simulink model "stm32f0_ccp_sensor"  (Simulink 7.3)
settings: Solver=ode3  SolverMode=SingleTasking  StartTime=0.0  StopTime=10.0  RelTol=1e-3
PreLoadFcn:
  | waijung.modelPreload; % Required for working with Waijung Blockset. Do not remove.
undefined symbols (not defined in the file): ARM, LQFP48, MDK, STM32F072CB
libraries: simulink x216, waijung_soft_i2c_lib x28, waijung_addon_module x12, stm32f0_flash_lib x10, stm32f0_can_lib x3, stm32f0_reset_lib x1, waijung_crc_lib x1, stm32f0_boot_lib x1, stm32f0_device_config_lib x1
(part 3 of 6)

== system stm32f0_ccp_sensor/HIH6131/Read/Subsystem ==
  In1 : Inport
  Enable : EnablePort
  Bitwise Operator : simulink/Logic and Bit Operations/Bitwise Operator  logicop=OR  UseBitMask=off  NumInputPorts=2  BitMask=bin2dec('11011001')  BitMaskRealWorld=Stored Integer
  Bitwise Operator1 : simulink/Logic and Bit Operations/Bitwise Operator  logicop=OR  UseBitMask=off  NumInputPorts=2  BitMask=bin2dec('11011001')  BitMaskRealWorld=Stored Integer
  Bitwise Operator2 : simulink/Logic and Bit Operations/Bitwise Operator  logicop=AND  UseBitMask=on  BitMask=hex2dec('3FFF')  BitMaskRealWorld=Stored Integer
  Bitwise Operator3 : simulink/Logic and Bit Operations/Bitwise Operator  logicop=AND  UseBitMask=on  BitMask=hex2dec('C000')  BitMaskRealWorld=Stored Integer
  Data Type Conversion : DataTypeConversion  OutDataTypeMode=uint16  OutDataType=fixdt(1, 16)  OutScaling=2^0  OutDataTypeStr=uint16
  Demux : Demux
  Shift Arithmetic : simulink/Logic and Bit Operations/Shift Arithmetic  SystemSampleTime=-1  nBitShiftRight=-8  nBinPtShiftRight=0
  Shift Arithmetic1 : simulink/Logic and Bit Operations/Shift Arithmetic  SystemSampleTime=-1  nBitShiftRight=-8  nBinPtShiftRight=0
  Shift Arithmetic2 : simulink/Logic and Bit Operations/Shift Arithmetic  SystemSampleTime=-1  nBitShiftRight=2  nBinPtShiftRight=0
  Shift Arithmetic3 : simulink/Logic and Bit Operations/Shift Arithmetic  SystemSampleTime=-1  nBitShiftRight=14  nBinPtShiftRight=0
  Status : Outport
  Humidity : Outport  Port=2
  Temperature : Outport  Port=3
  wires:
  Data Type Conversion/1 -> Demux/1
  Demux/1 -> Shift Arithmetic/1
  Shift Arithmetic/1 -> Bitwise Operator/1
  Demux/2 -> Bitwise Operator/2
  Demux/3 -> Shift Arithmetic1/1
  Shift Arithmetic1/1 -> Bitwise Operator1/1
  Demux/4 -> Bitwise Operator1/2
  Bitwise Operator/1 -> Bitwise Operator2/1, Bitwise Operator3/1
  Bitwise Operator1/1 -> Shift Arithmetic2/1
  Bitwise Operator3/1 -> Shift Arithmetic3/1
  Shift Arithmetic3/1 -> Status/1
  Bitwise Operator2/1 -> Humidity/1
  In1/1 -> Data Type Conversion/1
  Shift Arithmetic2/1 -> Temperature/1

== system stm32f0_ccp_sensor/MPL3115A2/MPL3115A2_Initialize/Write Configure ==
  note: # Priority 3
  note: # Priority 2
  note: # Priority 1
  SlvAddr : Inport  OutDataType=fixdt(1, 16)  OutScaling=2^0
  Enable : EnablePort
  PT_DATA_CFG : Constant  Value=hex2dec('13')  OutDataTypeMode=uint8  OutDataType=fixdt(1, 16)  OutScaling=2^0  OutDataTypeStr=uint8
  PT_DATA_CFG1 : Constant  Value=hex2dec('26')  OutDataTypeMode=uint8  OutDataType=fixdt(1, 16)  OutScaling=2^0  OutDataTypeStr=uint8
  PT_DATA_CFG2 : Constant  Value=hex2dec('26')  OutDataTypeMode=uint8  OutDataType=fixdt(1, 16)  OutScaling=2^0  OutDataTypeStr=uint8
  Soft I2C Master Read/Write : waijung_soft_i2c_lib/Soft I2C Master Read//Write  conf=ReadWrite  targetname=stm32f0  module=1  transfer=Blocking  clk=100  timeout=25  sdapins={'A4','A6'}  sclpins='A5'  writecount=2  readcount=0  waittime=0  forcestop=off  portpinstr=0  sampletime=inf  blockid=MPL3115A2MPL3115A2_InitializeWriteConfigureSoftI2CMasterReadWrite  inputporttype=[3 3 3]  inputportwidth=[]  inputportlabel={'SlvAddr' 'Wr0 (uint8)' 'Wr1 (uint8)'}  outputporttype=[3]  outputportwidth=[1]  outputportlabel={'Status'}  compat=0  optionstring="[\"1\",\"2\",\"0\",\"0\",\"off\",\"1\"]"
  Soft I2C Master Read/Write1 : waijung_soft_i2c_lib/Soft I2C Master Read//Write  conf=ReadWrite  targetname=stm32f0  module=1  transfer=Blocking  clk=100  timeout=25  sdapins={'A4','A6'}  sclpins='A5'  writecount=2  readcount=0  waittime=0  forcestop=off  portpinstr=0  sampletime=inf  blockid=MPL3115A2MPL3115A2_InitializeWriteConfigureSoftI2CMasterReadWrite1  inputporttype=[3 3 3]  inputportwidth=[]  inputportlabel={'SlvAddr' 'Wr0 (uint8)' 'Wr1 (uint8)'}  outputporttype=[3]  outputportwidth=[1]  outputportlabel={'Status'}  compat=0  optionstring="[\"1\",\"2\",\"0\",\"0\",\"off\",\"1\"]"
  Soft I2C Master Read/Write2 : waijung_soft_i2c_lib/Soft I2C Master Read//Write  conf=ReadWrite  targetname=stm32f0  module=1  transfer=Blocking  clk=100  timeout=25  sdapins={'A4','A6'}  sclpins='A5'  writecount=2  readcount=0  waittime=0  forcestop=off  portpinstr=0  sampletime=inf  blockid=MPL3115A2MPL3115A2_InitializeWriteConfigureSoftI2CMasterReadWrite2  inputporttype=[3 3 3]  inputportwidth=[]  inputportlabel={'SlvAddr' 'Wr0 (uint8)' 'Wr1 (uint8)'}  outputporttype=[3]  outputportwidth=[1]  outputportlabel={'Status'}  compat=0  optionstring="[\"1\",\"2\",\"0\",\"0\",\"off\",\"1\"]"
  Terminator : Terminator
  Terminator1 : Terminator
  Terminator2 : Terminator
  VAL : Constant  Value=7  OutDataTypeMode=uint8  OutDataType=fixdt(1, 16)  OutScaling=2^0  OutDataTypeStr=uint8
  VAL1 : Constant  Value=hex2dec('39')  OutDataTypeMode=uint8  OutDataType=fixdt(1, 16)  OutScaling=2^0  OutDataTypeStr=uint8
  VAL2 : Constant  Value=hex2dec('38')  OutDataTypeMode=uint8  OutDataType=fixdt(1, 16)  OutScaling=2^0  OutDataTypeStr=uint8
  wires:
  Soft I2C Master Read/Write2/1 -> Terminator2/1
  VAL1/1 -> Soft I2C Master Read/Write2/3
  PT_DATA_CFG2/1 -> Soft I2C Master Read/Write2/2
  Soft I2C Master Read/Write/1 -> Terminator1/1
  VAL2/1 -> Soft I2C Master Read/Write/3
  PT_DATA_CFG1/1 -> Soft I2C Master Read/Write/2
  Soft I2C Master Read/Write1/1 -> Terminator/1
  VAL/1 -> Soft I2C Master Read/Write1/3
  SlvAddr/1 -> Soft I2C Master Read/Write1/1, Soft I2C Master Read/Write2/1, Soft I2C Master Read/Write/1
  PT_DATA_CFG/1 -> Soft I2C Master Read/Write1/2

== system stm32f0_ccp_sensor/Network/Interface Configuration/CAN_ID Configuration/Enabled Subsystem ==
  In1 : Inport  OutDataType=fixdt(1, 16)  OutScaling=2^0
  Enable : EnablePort
  EEP Emulation Read : S-Function  Priority=1  FunctionName=stm32f0_eep_emulation  Parameters=conf,inputporttype,inputportwidth,outputporttype,outputportwidth,eepfilename,eepinfo,varname,optionstring,sampletime,blockid  EnableBusSupport=off  mask(stm32f0_eep_emulation){conf=Read, datatype=single, storagedefinename='Data1,Data2', storagename=CAN_ID, varname='CAN_ID', initialvalue=[1.0 2.0], storageindex=0, eepfilename='stm32f0_ccp_sensor.eeprom', eepinfo='CAN_ID,7,0,-', debuginfo=off, sampletime=inf, enablecustomportlabel=off, cinputportlabel=0, coutputportlabel=, portpinstr=0, blockid=NetworkInterfaceConfigurationCAN_IDConfigurationEnabledSubsystemEEPEmulationRead, inputporttype=[], inputportwidth=[], inputportlabel={}, outputporttype=[7], outputportwidth=[], outputportlabel={'CAN_ID'}, compat=0, optionstring=["CAN_ID","0","7","off","","","","","","","2","CAN_ID","7","0","dummy","0","0"]}
      mask prompts: conf "Configuration"; datatype "Storage type"; storagedefinename "Storage name"; storagename "Storage name"; varname "Var name (hidden)"; initialvalue "Initial value"; storageindex "Storage name index (hidden)"; eepfilename "EEP file name (hidden)"; eepinfo "EEP Information (hidden), [name, initialvalue, datatype]"; debuginfo "Debug information"; sampletime "Sample time (sec)"; enablecustomportlabel "Enable custom port labels (Ex. In1, In2, In3)"; cinputportlabel "Custom input port labels (Ex. In1, In2, In3)"; coutputportlabel "Custom output port labels (Ex. Out1, Out2, Out3)"; portpinstr "Port Pin String"; blockid "Block ID"; inputporttype "Input Port Type"; inputportwidth "Input Port Width"; inputportlabel "Input Port Label"; outputporttype "Output Port Type"; outputportwidth "Output Port Width"; outputportlabel "Output port label"; compat "Compatibility (Reserved for future use)"; optionstring "String(s) to be passed to TLC"
      mask help: Read a value from EEProm Emulation of the specified variable anme.
      mask init:
      | stm32f0_eep_emulation_callback('init');
      mask Help: web(fullfile(waijungdocroot,'stm32f0_eep_emulation_read.htm'), '-browser')
      mask StyleString: popup(Setup|Read|Write),popup(double|single|int8|uint8|int16|uint16|int32|uint32),edit,popup(CAN_ID),edit,edit,edit,edit,edit,checkbox,edit,checkbox,edit,edit,edit,edit,edit,edit,edit,edit,edit,edit,edit,edit
      mask CallbackString: stm32f0_eep_emulation_callback('conf');||stm32f0_eep_emulation_callback('storagedefinename');||stm32f0_eep_emulation_callback('varname');|||stm32f0_eep_emulation_callback('eepfilename');||stm32f0_eep_emulation_callback('debuginfo');|stm32f0_eep_emulation_callback('sampletime');|stm32f0_eep_emulation_callback('enablecustomportlabel');|stm32f0_eep_emulation_callback('conf');|stm32f0_eep_emulation_callback('conf');||stm32f0_eep_emulation_callback('blockid');||||||||
      mask Display: text(0.5, 0.5, '[EEP Read]\nName: CAN_ID\nTs (sec): 0.01','ver','middle','hor','center'); port_label('output', 1,'CAN_ID');
  EEP Emulation Write : S-Function  Priority=0  FunctionName=stm32f0_eep_emulation  Parameters=conf,inputporttype,inputportwidth,outputporttype,outputportwidth,eepfilename,eepinfo,varname,optionstring,sampletime,blockid  EnableBusSupport=off  mask(stm32f0_eep_emulation){conf=Write, datatype=single, storagedefinename='Data1,Data2', storagename=CAN_ID, varname='CAN_ID', initialvalue=[1.0 2.0], storageindex=0, eepfilename='stm32f0_ccp_sensor.eeprom', eepinfo='CAN_ID,7,0,-', debuginfo=off, sampletime=inf, enablecustomportlabel=off, cinputportlabel=0, coutputportlabel=, portpinstr=0, blockid=NetworkInterfaceConfigurationCAN_IDConfigurationEnabledSubsystemEEPEmulationWrite, inputporttype=[-1], inputportwidth=[], inputportlabel={'CAN_ID'}, outputporttype=[], outputportwidth=[], outputportlabel={}, compat=0, optionstring=["CAN_ID","0","7","off","","","","","","","2","CAN_ID","7","0","dummy","0","0"]}
      mask prompts: conf "Configuration"; datatype "Storage type"; storagedefinename "Storage name"; storagename "Storage name"; varname "Var name (hidden)"; initialvalue "Initial value"; storageindex "Storage name index (hidden)"; eepfilename "EEP file name (hidden)"; eepinfo "EEP Information (hidden), [name, initialvalue, datatype]"; debuginfo "Debug information"; sampletime "Sample time (sec)"; enablecustomportlabel "Enable custom port labels (Ex. In1, In2, In3)"; cinputportlabel "Custom input port labels (Ex. In1, In2, In3)"; coutputportlabel "Custom output port labels (Ex. Out1, Out2, Out3)"; portpinstr "Port Pin String"; blockid "Block ID"; inputporttype "Input Port Type"; inputportwidth "Input Port Width"; inputportlabel "Input Port Label"; outputporttype "Output Port Type"; outputportwidth "Output Port Width"; outputportlabel "Output port label"; compat "Compatibility (Reserved for future use)"; optionstring "String(s) to be passed to TLC"
      mask help: Write data value to the specified variable name, to store in EEProm Emulation.
      mask init:
      | stm32f0_eep_emulation_callback('init');
      mask Help: web(fullfile(waijungdocroot,'stm32f0_eep_emulation_write.htm'), '-browser')
      mask StyleString: popup(Setup|Read|Write),popup(double|single|int8|uint8|int16|uint16|int32|uint32),edit,popup(CAN_ID),edit,edit,edit,edit,edit,checkbox,edit,checkbox,edit,edit,edit,edit,edit,edit,edit,edit,edit,edit,edit,edit
      mask CallbackString: stm32f0_eep_emulation_callback('conf');||stm32f0_eep_emulation_callback('storagedefinename');||stm32f0_eep_emulation_callback('varname');|||stm32f0_eep_emulation_callback('eepfilename');||stm32f0_eep_emulation_callback('debuginfo');|stm32f0_eep_emulation_callback('sampletime');|stm32f0_eep_emulation_callback('enablecustomportlabel');|stm32f0_eep_emulation_callback('conf');|stm32f0_eep_emulation_callback('conf');||stm32f0_eep_emulation_callback('blockid');||||||||
      mask Display: text(0.5, 0.5, '[EEP Write]\nName: CAN_ID\nTs (sec): 0.01','ver','middle','hor','center'); port_label('input', 1,'CAN_ID');
  UART Tx : S-Function  FunctionName=stm32f0_uart  Parameters=conf,inputporttype,inputportwidth,outputporttype,outputportwidth,asciiheader,optionstring,headerstring,terminatorstring,asciidatatypestring,sampletime,blockid  EnableBusSupport=off  mask(stm32f0_uart){conf=Tx, uartmodule=1, baudrate=115200, databits=8, parity=No, stopbit=1, remaptxpin=A9, remaprxpin=A10, flowcontrol=None, remapctspin=Not used, remaprtspin=Not used, advanceoptions=off, rxbuffersize=64, txbuffersize=64, transfer=Non-Blocking, packetmode=Ascii, binheader='7E 7E', binterminator='03 03', porttype_double=0, porttype_single=0, porttype_int8=0, porttype_uint8=0, porttype_int16=0, porttype_uint16=0, porttype_int32=0, porttype_uint32=2, asciiformat='Ok, id=%u', rx_asciiterminator=CR (0x0D - "\r"), tx_asciiterminator=CRLF (0x0D 0x0A - "\r\n"), storagename=<empty>, varname=, asciiheader=Ok, id=%u\r\n, sampletime=inf, enablecustomportlabel=off, cinputportlabel=de, coutputportlabel=fff,ff,sdfsd, portpinstr=0, blockid=NetworkInterfaceConfigurationCAN_IDConfigurationEnabledSubsystemUARTTx, inputporttype=[ -1], inputportwidth=[], inputportlabel={ '%u'}, outputporttype=[], outputportwidth=[], outputportlabel={}, compat=0, optionstring=["1", "1", "A", "9", "1", "A", "10", "0", "*", "*", "0", "*", "*", "1", "1", "", "", "115200", "8", "No", "1", "None", "3", "2", "64", "64", "Ascii", "Non-Blocking", ""], headerstring=[], terminatorstring=["13","10"], asciidatatypestring=["uint32_t"], lastmodule=1}
      mask prompts: conf "Configuration"; uartmodule "UART Module"; baudrate "Baud rate (bps)"; databits "Data bits"; stopbit "Stop bit"; remaptxpin "Tx pin"; remaprxpin "Rx pin"; flowcontrol "Hardware flow control"; remapctspin "HW Flow control, CTS Pin"; remaprtspin "HW Flow control, RTS Pin"; advanceoptions "Advance options"; rxbuffersize "Rx buffer size (bytes)"; txbuffersize "Tx buffer size (bytes)"; packetmode "Packet mode"; binheader "Binary header (example: '7E 7E')"; binterminator "Binary terminator (example: '03 03')"; porttype_double "Number of data port, type DOUBLE"; porttype_single "Number of data port, type SINGLE"; porttype_int8 "Number of data port, type INT8"; porttype_uint8 "Number of data port, type UINT8"; porttype_int16 "Number of data port, type INT16"; porttype_uint16 "Number of data port, type UINT16"; porttype_int32 "Number of data port, type INT32"; porttype_uint32 "Number of data port, type UINT32"; asciiformat "Ascii format"; rx_asciiterminator "End of packet"; tx_asciiterminator "End of packet"; storagename "Buffer"; varname "Var name"; asciiheader "Ascii header (printf format)"; sampletime "Sample time (sec)"; enablecustomportlabel "Enable custom port labels (Ex. In1, In2, In3)"; cinputportlabel "Custom input port labels (Ex. In1, In2, In3)"; coutputportlabel "Custom output port labels (Ex. Out1, Out2, Out3)"; portpinstr "Port Pin String"; blockid "Block ID"; inputporttype "Input Port Type"; inputportwidth "Input Port Width"; inputportlabel "Input Port Label"; outputporttype "Output Port Type"; outputportwidth "Output Port Width"; outputportlabel "Output port label"; compat "Compatibility (Reserved for future use)"; optionstring "String(s) to be passed to TLC"; lastmodule "Last module selected"
      mask help:
      | UART Module
      |  - Select module corresponding to "UART Setup" block.
      | Transfer
      |  - Blocking: after write DMA buffer, the block wait until buffer empty.
      |  - Non-Blocking: the block will not wait for buffer empty.
      | Packet mode:
      |  - Ascii: sending data is ascii, Ascii format + End of packet.
      |  - Binary: sending data is binary format, Header + Data + Terminator
      |  - String Buffer: Volatile Data Storage variable name as sending data.
      | Ascii format:
      |  - %U, %I, %D, %O, %X, %u, %i, %d, %o, %x: Uint32
      |  - %E, %G, %F, %e, %g, %f: Single
      |  - %C, %c: Int8
      |  - %S, %s: (char *), this port is output of Volatile Data Storage Read block, which data type is string.
      mask init:
      | stm32f0_uart_callback('init');
      mask Help: web(fullfile(waijungdocroot,'stm32f0_uart_tx.htm'), '-browser')
      mask StyleString: popup(Setup|Tx|Rx),popup(1|2|3|4),edit,popup(8),popup(No|Odd|Even),popup(0.5|1|1.5|2),popup(Not used|A9|B6),popup(Not used|A10|B7),popup(None|RTS|CTS|RTS/CTS),popup(Not used|A11),popup(Not used|A12),checkbox,popup(16|32|64|128|256|512),popup(16|32|64|128|256|512),popup(Blocking|Non-Blocking),popup(Ascii|Binary|String Buffer),edit,edit,edit,edit,edit,edit,edit,edit,edit,edit,edit,popup(CR (0x0D - "\r")|LF (0x0A - "\n")|CRLF (0x0D 0x0A - "\r\n")),popup(CR (0x0D - "\r")|LF (0x0A - "\n")|CRLF (0x0D 0x0A - "\r\n")|None),popup(<empty>),edit,edit,edit,checkbox,edit,edit,edit,edit,edit,edit,edit,edit,edit,edit,edit,edit,edit,edit,edit,edit
      mask CallbackString: stm32f0_uart_callback('conf');|stm32f0_uart_callback('uartmodule');|||||||stm32f0_uart_callback('flowcontrol');|||stm32f0_uart_callback('advanceoptions');|||stm32f0_uart_callback('conf');|stm32f0_uart_callback('conf');|stm32f0_uart_callback('binheader');|stm32f0_uart_callback('binterminator');|||||||||stm32f0_uart_callback('asciiformat');|||stm32f0_uart_callback('storagename');|||stm32f0_uart_callback('sampletime');|stm32f0_uart_callback('enablecustomportlabel');|stm32f0_uart_callback('conf');|stm32f0_uart_callback('conf');||stm32f0_uart_callback('blockid');||||||||||||
      mask Display: text(0.95, 0.5, 'Module: USART1_Tx\nPacket: Ascii\nTransfer: Non-Blocking\nTs (sec): 0.01','ver','middle','hor','right'); port_label('input', 1,'%u');
  wires:
  In1/1 -> EEP Emulation Write/1
  EEP Emulation Read/1 -> UART Tx/1

== system stm32f0_ccp_sensor/CCP Handler/CRO CONNECT Parser/CONNECT Handler/Enabled Subsystem ==
  CMD : Inport  OutDataType=fixdt(1, 16)  OutScaling=2^0
  Station address Lsb : Inport  Port=2  OutDataType=fixdt(1, 16)  OutScaling=2^0
  Station address Msb : Inport  Port=3  OutDataType=fixdt(1, 16)  OutScaling=2^0
  Enable : EnablePort
  CONNECT : simulink/Logic and Bit Operations/Compare To Constant  SystemSampleTime=-1  relop===  const=1  LogicOutDataTypeMode=uint8  ZeroCross=off
  DISCONNECT : simulink/Logic and Bit Operations/Compare To Constant  SystemSampleTime=-1  relop===  const=7  LogicOutDataTypeMode=uint8  ZeroCross=off
  Enabled Subsystem : Subsystem  TreatAsAtomicUnit=on
  Logical Operator : Logic  Operator=OR  AllPortsSameDT=off  OutDataTypeMode=boolean  LogicDataType=fixdt(0, 8)  OutDataTypeStr=boolean
  Connected : Outport  OutDataType=fixdt(1, 16)  OutScaling=2^0
  Station Addr : Outport  Port=2  OutDataType=fixdt(1, 16)  OutScaling=2^0
  wires:
  CMD/1 -> CONNECT/1, DISCONNECT/1
  CONNECT/1 -> Enabled Subsystem/Enable, Logical Operator/2
  Station address Lsb/1 -> Enabled Subsystem/1(In1)
  Enabled Subsystem/1(Out1) -> Station Addr/1
  Station address Msb/1 -> Enabled Subsystem/2(In2)
  Logical Operator/1 -> Connected/1
  DISCONNECT/1 -> Logical Operator/1

== system stm32f0_ccp_sensor/CCP Handler/CRO MTA Parser/Enabled Subsystem/Convert ==
  ExtAddr : Inport  OutDataType=fixdt(1, 16)  OutScaling=2^0
  In1 : Inport  Port=2  OutDataType=fixdt(1, 16)  OutScaling=2^0
  In2 : Inport  Port=3  OutDataType=fixdt(1, 16)  OutScaling=2^0
  In3 : Inport  Port=4  OutDataType=fixdt(1, 16)  OutScaling=2^0
  In4 : Inport  Port=5  OutDataType=fixdt(1, 16)  OutScaling=2^0
  Enable : EnablePort
  Bitwise Operator : simulink/Logic and Bit Operations/Bitwise Operator  logicop=OR  UseBitMask=off  NumInputPorts=4  BitMask=bin2dec('11011001')  BitMaskRealWorld=Stored Integer
  Data Type Conversion{,1..3} (4 alike) : DataTypeConversion  OutDataTypeMode=uint32  OutDataType=fixdt(1, 16)  OutScaling=2^0  OutDataTypeStr=uint32
  Shift Arithmetic : simulink/Logic and Bit Operations/Shift Arithmetic  SystemSampleTime=-1  nBitShiftRight=-16  nBinPtShiftRight=0
  Shift Arithmetic1 : simulink/Logic and Bit Operations/Shift Arithmetic  SystemSampleTime=-1  nBitShiftRight=-8  nBinPtShiftRight=0
  Shift Arithmetic3 : simulink/Logic and Bit Operations/Shift Arithmetic  SystemSampleTime=-1  nBitShiftRight=-24  nBinPtShiftRight=0
  ExtAddt_out : Outport  OutDataType=fixdt(1, 16)  OutScaling=2^0
  Address : Outport  Port=2  OutDataType=fixdt(1, 16)  OutScaling=2^0
  wires:
  In1/1 -> Data Type Conversion/1
  In2/1 -> Data Type Conversion1/1
  In3/1 -> Data Type Conversion2/1
  In4/1 -> Data Type Conversion3/1
  Data Type Conversion3/1 -> Bitwise Operator/4
  Data Type Conversion2/1 -> Shift Arithmetic1/1
  Data Type Conversion/1 -> Shift Arithmetic3/1
  Shift Arithmetic1/1 -> Bitwise Operator/3
  Bitwise Operator/1 -> Address/1
  Shift Arithmetic3/1 -> Bitwise Operator/1
  Data Type Conversion1/1 -> Shift Arithmetic/1
  Shift Arithmetic/1 -> Bitwise Operator/2
  ExtAddr/1 -> ExtAddt_out/1

== system stm32f0_ccp_sensor/CCP Handler/CRO UNLOCK Parser/Enabled Subsystem/Enabled Subsystem ==
  In1 : Inport  OutDataType=fixdt(1, 16)  OutScaling=2^0
  Last state : Inport  Port=2  OutDataType=fixdt(1, 16)  OutScaling=2^0
  Enable : EnablePort
  CAL_KEY : Constant  Value=[0 0 10 10 10 10]  OutDataTypeMode=uint8  OutDataType=fixdt(1, 16)  OutScaling=2^0  OutDataTypeStr=uint8
  DAQ_KEY : Constant  Value=[0 0 12 12 12 12]  OutDataTypeMode=uint8  OutDataType=fixdt(1, 16)  OutScaling=2^0  OutDataTypeStr=uint8
  Demux : Demux  Outputs=3
  Mux : Mux  Inputs=3
  PGM_KEY : Constant  Value=[0 0 11 11 11 11]  OutDataTypeMode=uint8  OutDataType=fixdt(1, 16)  OutScaling=2^0  OutDataTypeStr=uint8
  Subsystem : Subsystem
  Subsystem1 : Subsystem
  Subsystem2 : Subsystem
  Switch : Switch  Criteria=u2 > Threshold  OutDataType=fixdt(1, 16)  OutScaling=2^0
  Switch1 : Switch  Criteria=u2 > Threshold  OutDataType=fixdt(1, 16)  OutScaling=2^0
  Switch2 : Switch  Criteria=u2 > Threshold  OutDataType=fixdt(1, 16)  OutScaling=2^0
  Unlocked : Constant  OutDataTypeMode=uint8  OutDataType=fixdt(1, 16)  OutScaling=2^0  OutDataTypeStr=uint8
  Out1 : Outport  OutDataType=fixdt(1, 16)  OutScaling=2^0
  wires:
  Mux/1 -> Out1/1
  CAL_KEY/1 -> Subsystem/1(In1)
  In1/1 -> Subsystem/2(In2), Subsystem1/2(In2), Subsystem2/2(In2)
  Subsystem/1(Out1) -> Switch/2
  PGM_KEY/1 -> Subsystem1/1(In1)
  Subsystem1/1(Out1) -> Switch1/2
  DAQ_KEY/1 -> Subsystem2/1(In1)
  Subsystem2/1(Out1) -> Switch2/2
  Last state/1 -> Demux/1
  Demux/1 -> Switch/3
  Demux/2 -> Switch1/3
  Demux/3 -> Switch2/3
  Unlocked/1 -> Switch/1, Switch1/1, Switch2/1
  Switch1/1 -> Mux/2
  Switch/1 -> Mux/1
  Switch2/1 -> Mux/3

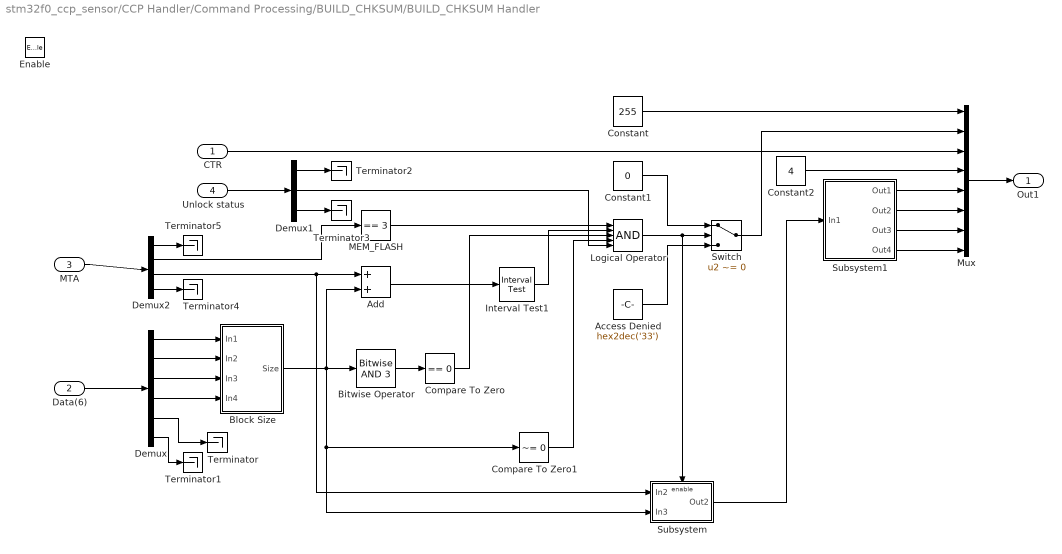
== system stm32f0_ccp_sensor/CCP Handler/Command Processing/BUILD_CHKSUM/BUILD_CHKSUM Handler ==
  CTR : Inport  OutDataType=fixdt(1, 16)  OutScaling=2^0
  Data(6) : Inport  Port=2
  MTA : Inport  Port=3
  Unlock status : Inport  Port=4
  Enable : EnablePort
  Access Denied : Constant  Value=hex2dec('33')  OutDataTypeMode=uint8  OutDataType=fixdt(1, 16)  OutScaling=2^0  OutDataTypeStr=uint8
  Add : Sum  OutDataType=fixdt(1, 16)  OutScaling=2^-10
  Bitwise Operator : simulink/Logic and Bit Operations/Bitwise Operator  logicop=AND  UseBitMask=on  BitMask=3  BitMaskRealWorld=Stored Integer
  Block Size : Subsystem
  Compare To Zero : simulink/Logic and Bit Operations/Compare To Zero  SystemSampleTime=-1  relop===  LogicOutDataTypeMode=uint8  ZeroCross=off
  Compare To Zero1 : simulink/Logic and Bit Operations/Compare To Zero  SystemSampleTime=-1  relop=~=  LogicOutDataTypeMode=uint8  ZeroCross=off
  Constant : Constant  Value=255  OutDataTypeMode=uint8  OutDataType=fixdt(1, 16)  OutScaling=2^0  OutDataTypeStr=uint8
  Constant1 : Constant  Value=0  OutDataTypeMode=uint8  OutDataType=fixdt(1, 16)  OutScaling=2^0  OutDataTypeStr=uint8
  Constant2 : Constant  Value=4  OutDataTypeMode=uint8  OutDataType=fixdt(1, 16)  OutScaling=2^0  OutDataTypeStr=uint8
  Demux : Demux  Outputs=6
  Demux1 : Demux  Outputs=3
  Demux2 : Demux
  Interval Test1 : simulink/Logic and Bit Operations/Interval Test  SystemSampleTime=-1  IntervalClosedRight=on  uplimit=52*1024  IntervalClosedLeft=on  lowlimit=0  LogicOutDataTypeMode=boolean
  Logical Operator : Logic  Inputs=5  AllPortsSameDT=off  OutDataTypeMode=boolean  LogicDataType=fixdt(0, 8)  OutDataTypeStr=boolean
  MEM_FLASH : simulink/Logic and Bit Operations/Compare To Constant  SystemSampleTime=-1  relop===  const=3  LogicOutDataTypeMode=uint8  ZeroCross=off
  Mux : Mux  Inputs=8
  Subsystem : Subsystem
  Subsystem1 : Subsystem
  Switch : Switch  Criteria=u2 ~= 0  OutDataType=fixdt(1, 16)  OutScaling=2^0
  Terminator{,1..5} (6 alike) : Terminator
  Out1 : Outport  OutDataType=fixdt(1, 16)  OutScaling=2^0  InitialOutput=[0 0 0 0 0 0 0 0]
  wires:
  Mux/1 -> Out1/1
  Constant/1 -> Mux/1
  CTR/1 -> Mux/3
  Data(6)/1 -> Demux/1
  Demux/1 -> Block Size/1(In1)
  Demux/2 -> Block Size/2(In2)
  Demux/3 -> Block Size/3(In3)
  Demux/4 -> Block Size/4(In4)
  Demux/5 -> Terminator/1
  Demux/6 -> Terminator1/1
  Block Size/1(Size) -> Add/2, Bitwise Operator/1, Compare To Zero1/1, Subsystem/2(In3)
  Add/1 -> Interval Test1/1
  Interval Test1/1 -> Logical Operator/2
  Bitwise Operator/1 -> Compare To Zero/1
  Compare To Zero/1 -> Logical Operator/3
  Logical Operator/1 -> Switch/2, Subsystem/Enable
  Switch/1 -> Mux/2
  Constant1/1 -> Switch/1
  Access Denied/1 -> Switch/3
  Constant2/1 -> Mux/4
  Compare To Zero1/1 -> Logical Operator/4
  Subsystem1/1(Out1) -> Mux/5
  Subsystem1/2(Out2) -> Mux/6
  Subsystem1/3(Out3) -> Mux/7
  Subsystem1/4(Out4) -> Mux/8
  Subsystem/1(Out2) -> Subsystem1/1(In1)
  Unlock status/1 -> Demux1/1
  Demux1/2 -> Logical Operator/5
  Demux1/1 -> Terminator2/1
  Demux1/3 -> Terminator3/1
  MTA/1 -> Demux2/1
  Demux2/2 -> MEM_FLASH/1
  MEM_FLASH/1 -> Logical Operator/1
  Demux2/3 -> Add/1, Subsystem/1(In2)
  Demux2/4 -> Terminator4/1
  Demux2/1 -> Terminator5/1

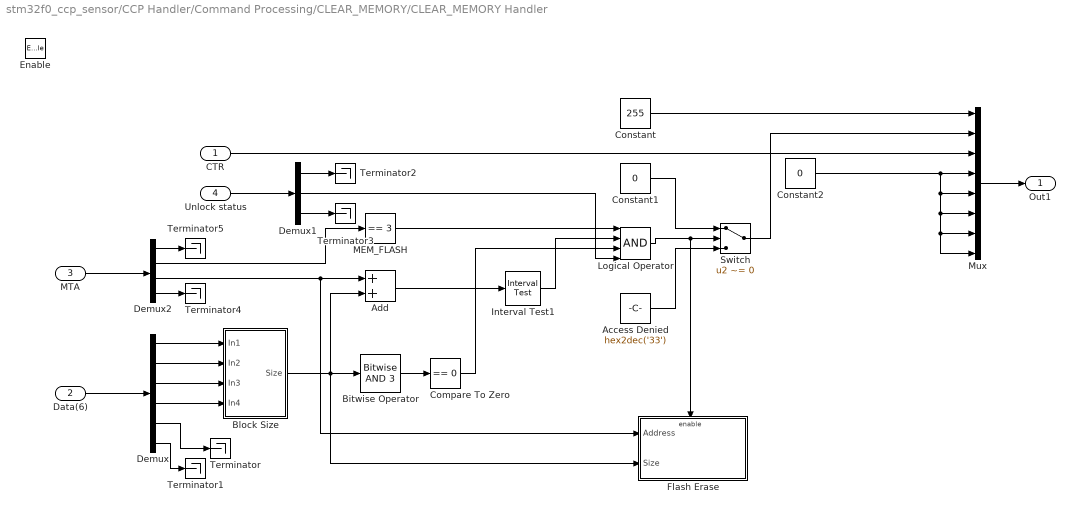
== system stm32f0_ccp_sensor/CCP Handler/Command Processing/CLEAR_MEMORY/CLEAR_MEMORY Handler ==
  CTR : Inport  OutDataType=fixdt(1, 16)  OutScaling=2^0
  Data(6) : Inport  Port=2
  MTA : Inport  Port=3
  Unlock status : Inport  Port=4
  Enable : EnablePort
  Access Denied : Constant  Value=hex2dec('33')  OutDataTypeMode=uint8  OutDataType=fixdt(1, 16)  OutScaling=2^0  OutDataTypeStr=uint8
  Add : Sum  OutDataType=fixdt(1, 16)  OutScaling=2^-10
  Bitwise Operator : simulink/Logic and Bit Operations/Bitwise Operator  logicop=AND  UseBitMask=on  BitMask=3  BitMaskRealWorld=Stored Integer
  Block Size : Subsystem
  Compare To Zero : simulink/Logic and Bit Operations/Compare To Zero  SystemSampleTime=-1  relop===  LogicOutDataTypeMode=uint8  ZeroCross=off
  Constant : Constant  Value=255  OutDataTypeMode=uint8  OutDataType=fixdt(1, 16)  OutScaling=2^0  OutDataTypeStr=uint8
  Constant1 : Constant  Value=0  OutDataTypeMode=uint8  OutDataType=fixdt(1, 16)  OutScaling=2^0  OutDataTypeStr=uint8
  Constant2 : Constant  Value=0  OutDataTypeMode=uint8  OutDataType=fixdt(1, 16)  OutScaling=2^0  OutDataTypeStr=uint8
  Demux : Demux  Outputs=6
  Demux1 : Demux  Outputs=3
  Demux2 : Demux
  Flash Erase : Subsystem
  Interval Test1 : simulink/Logic and Bit Operations/Interval Test  SystemSampleTime=-1  IntervalClosedRight=on  uplimit=52*1024  IntervalClosedLeft=on  lowlimit=2  LogicOutDataTypeMode=boolean
  Logical Operator : Logic  Inputs=4  AllPortsSameDT=off  OutDataTypeMode=boolean  LogicDataType=fixdt(0, 8)  OutDataTypeStr=boolean
  MEM_FLASH : simulink/Logic and Bit Operations/Compare To Constant  SystemSampleTime=-1  relop===  const=3  LogicOutDataTypeMode=uint8  ZeroCross=off
  Mux : Mux  Inputs=8
  Switch : Switch  Criteria=u2 ~= 0  OutDataType=fixdt(1, 16)  OutScaling=2^0
  Terminator{,1..5} (6 alike) : Terminator
  Out1 : Outport  OutDataType=fixdt(1, 16)  OutScaling=2^0  InitialOutput=[0 0 0 0 0 0 0 0]
  wires:
  Mux/1 -> Out1/1
  Constant/1 -> Mux/1
  CTR/1 -> Mux/3
  Data(6)/1 -> Demux/1
  Demux/1 -> Block Size/1(In1)
  Demux/2 -> Block Size/2(In2)
  Demux/3 -> Block Size/3(In3)
  Demux/4 -> Block Size/4(In4)
  Demux/5 -> Terminator/1
  Demux/6 -> Terminator1/1
  Block Size/1(Size) -> Add/2, Bitwise Operator/1, Flash Erase/2(Size)
  Add/1 -> Interval Test1/1
  Interval Test1/1 -> Logical Operator/2
  Bitwise Operator/1 -> Compare To Zero/1
  Compare To Zero/1 -> Logical Operator/3
  Logical Operator/1 -> Switch/2, Flash Erase/Enable
  Switch/1 -> Mux/2
  Constant1/1 -> Switch/1
  Access Denied/1 -> Switch/3
  Constant2/1 -> Mux/4, Mux/5, Mux/6, Mux/7, Mux/8
  Unlock status/1 -> Demux1/1
  Demux1/2 -> Logical Operator/4
  Demux1/1 -> Terminator2/1
  Demux1/3 -> Terminator3/1
  MTA/1 -> Demux2/1
  Demux2/2 -> MEM_FLASH/1
  MEM_FLASH/1 -> Logical Operator/1
  Demux2/3 -> Add/1, Flash Erase/1(Address)
  Demux2/4 -> Terminator4/1
  Demux2/1 -> Terminator5/1

== system stm32f0_ccp_sensor/CCP Handler/Command Processing/CONNECT/CONNECT Handler ==
  CTR : Inport  OutDataType=fixdt(1, 16)  OutScaling=2^0
  Enable : EnablePort
  Constant : Constant  Value=255  OutDataTypeMode=uint8  OutDataType=fixdt(1, 16)  OutScaling=2^0  OutDataTypeStr=uint8
  Constant1 : Constant  Value=0  OutDataTypeMode=uint8  OutDataType=fixdt(1, 16)  OutScaling=2^0  OutDataTypeStr=uint8
  Mux : Mux  Inputs=8
  Out1 : Outport  OutDataType=fixdt(1, 16)  OutScaling=2^0  InitialOutput=[0 0 0 0 0 0 0 0]
  wires:
  CTR/1 -> Mux/3
  Constant/1 -> Mux/1
  Constant1/1 -> Mux/4, Mux/2, Mux/5, Mux/6, Mux/7, Mux/8
  Mux/1 -> Out1/1

== system stm32f0_ccp_sensor/CCP Handler/Command Processing/DISCONNECT/DISCONNECT Handler ==
  CTR : Inport  OutDataType=fixdt(1, 16)  OutScaling=2^0
  Unlock status : Inport  Port=2  OutDataType=fixdt(1, 16)  OutScaling=2^0
  Enable : EnablePort
  Constant : Constant  Value=255  OutDataTypeMode=uint8  OutDataType=fixdt(1, 16)  OutScaling=2^0  OutDataTypeStr=uint8
  Constant1 : Constant  Value=0  OutDataTypeMode=uint8  OutDataType=fixdt(1, 16)  OutScaling=2^0  OutDataTypeStr=uint8
  Demux : Demux  Outputs=3
  Mux : Mux  Inputs=8
  Terminator : Terminator
  Terminator1 : Terminator
  Out1 : Outport  OutDataType=fixdt(1, 16)  OutScaling=2^0  InitialOutput=[0 0 0 0 0 0 0 0]
  Reset : Outport  Port=2  OutDataType=fixdt(1, 16)  OutScaling=2^0  InitialOutput=0
  wires:
  Mux/1 -> Out1/1
  Constant1/1 -> Mux/8, Mux/7, Mux/6, Mux/5, Mux/2, Mux/4
  Constant/1 -> Mux/1
  CTR/1 -> Mux/3
  Demux/2 -> Reset/1
  Demux/1 -> Terminator/1
  Demux/3 -> Terminator1/1
  Unlock status/1 -> Demux/1

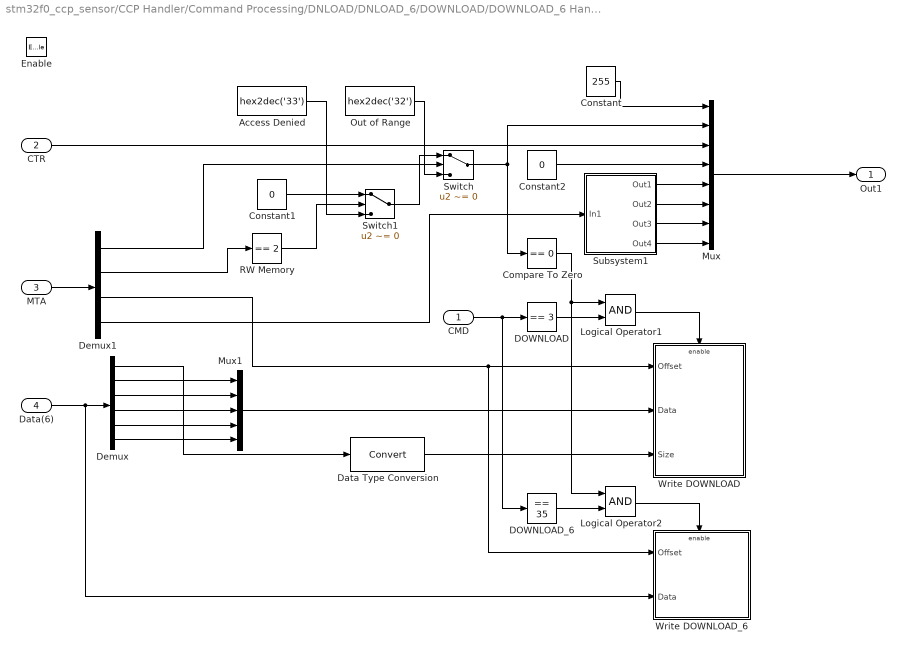
== system stm32f0_ccp_sensor/CCP Handler/Command Processing/DNLOAD/DNLOAD_6/DOWNLOAD/DOWNLOAD_6 Handler ==
  CMD : Inport  OutDataType=fixdt(1, 16)  OutScaling=2^0
  CTR : Inport  Port=2  OutDataType=fixdt(1, 16)  OutScaling=2^0
  MTA : Inport  Port=3  OutDataType=fixdt(1, 16)  OutScaling=2^0
  Data(6) : Inport  Port=4  OutDataType=fixdt(1, 16)  OutScaling=2^0
  Enable : EnablePort
  Access Denied : Constant  Value=hex2dec('33')  OutDataTypeMode=uint8  OutDataType=fixdt(1, 16)  OutScaling=2^0  OutDataTypeStr=uint8
  Compare To Zero : simulink/Logic and Bit Operations/Compare To Zero  SystemSampleTime=-1  relop===  LogicOutDataTypeMode=uint8  ZeroCross=off
  Constant : Constant  Value=255  OutDataTypeMode=uint8  OutDataType=fixdt(1, 16)  OutScaling=2^0  OutDataTypeStr=uint8
  Constant1 : Constant  Value=0  OutDataTypeMode=uint8  OutDataType=fixdt(1, 16)  OutScaling=2^0  OutDataTypeStr=uint8
  Constant2 : Constant  Value=0  OutDataTypeMode=uint8  OutDataType=fixdt(1, 16)  OutScaling=2^0  OutDataTypeStr=uint8
  DOWNLOAD : simulink/Logic and Bit Operations/Compare To Constant  SystemSampleTime=-1  relop===  const=3  LogicOutDataTypeMode=uint8  ZeroCross=off
  DOWNLOAD_6 : simulink/Logic and Bit Operations/Compare To Constant  SystemSampleTime=-1  relop===  const=35  LogicOutDataTypeMode=uint8  ZeroCross=off
  Data Type Conversion : DataTypeConversion  OutDataType=fixdt(1, 16)  OutScaling=2^0
  Demux : Demux  Outputs=6
  Demux1 : Demux
  Logical Operator1 : Logic  AllPortsSameDT=off  OutDataTypeMode=boolean  LogicDataType=fixdt(0, 8)  OutDataTypeStr=boolean
  Logical Operator2 : Logic  AllPortsSameDT=off  OutDataTypeMode=boolean  LogicDataType=fixdt(0, 8)  OutDataTypeStr=boolean
  Mux : Mux  Inputs=8
  Mux1 : Mux  Inputs=5
  Out of Range : Constant  Value=hex2dec('32')  OutDataTypeMode=uint8  OutDataType=fixdt(1, 16)  OutScaling=2^0  OutDataTypeStr=uint8
  RW Memory : simulink/Logic and Bit Operations/Compare To Constant  SystemSampleTime=-1  relop===  const=2  LogicOutDataTypeMode=uint8  ZeroCross=off
  Subsystem1 : Subsystem
  Switch : Switch  Criteria=u2 ~= 0  OutDataType=fixdt(1, 16)  OutScaling=2^0
  Switch1 : Switch  Criteria=u2 ~= 0  OutDataType=fixdt(1, 16)  OutScaling=2^0
  Write DOWNLOAD : Subsystem
  Write DOWNLOAD_6 : Subsystem
  Out1 : Outport  OutDataType=fixdt(1, 16)  OutScaling=2^0  InitialOutput=[0 0 0 0 0 0 0 0]
  wires:
  Mux/1 -> Out1/1
  Constant/1 -> Mux/1
  CTR/1 -> Mux/3
  Data(6)/1 -> Demux/1, Write DOWNLOAD_6/2(Data)
  MTA/1 -> Demux1/1
  Demux/1 -> Data Type Conversion/1
  Switch1/1 -> Switch/1
  Constant1/1 -> Switch1/1
  Switch/1 -> Mux/2, Compare To Zero/1
  Demux1/3 -> Write DOWNLOAD/1(Offset), Write DOWNLOAD_6/1(Offset)
  Demux/2 -> Mux1/1
  Demux/3 -> Mux1/2
  Demux/4 -> Mux1/3
  Demux/5 -> Mux1/4
  Demux/6 -> Mux1/5
  Mux1/1 -> Write DOWNLOAD/2(Data)
  Constant2/1 -> Mux/4
  Subsystem1/1(Out1) -> Mux/5
  Subsystem1/2(Out2) -> Mux/6
  Subsystem1/3(Out3) -> Mux/7
  Subsystem1/4(Out4) -> Mux/8
  Data Type Conversion/1 -> Write DOWNLOAD/3(Size)
  Compare To Zero/1 -> Logical Operator1/1, Logical Operator2/1
  CMD/1 -> DOWNLOAD/1, DOWNLOAD_6/1
  DOWNLOAD/1 -> Logical Operator1/2
  Logical Operator1/1 -> Write DOWNLOAD/Enable
  Logical Operator2/1 -> Write DOWNLOAD_6/Enable
  DOWNLOAD_6/1 -> Logical Operator2/2
  Demux1/1 -> Switch/2
  Out of Range/1 -> Switch/3
  Demux1/2 -> RW Memory/1
  RW Memory/1 -> Switch1/2
  Access Denied/1 -> Switch1/3
  Demux1/4 -> Subsystem1/1(In1)

== system stm32f0_ccp_sensor/CCP Handler/Command Processing/EXCHANGE_ID/EXCHANGE_ID Handler ==
  CTR : Inport  OutDataType=fixdt(1, 16)  OutScaling=2^0
  Enable : EnablePort
  Constant : Constant  Value=255  OutDataTypeMode=uint8  OutDataType=fixdt(1, 16)  OutScaling=2^0  OutDataTypeStr=uint8
  Constant1 : Constant  Value=0  OutDataTypeMode=uint8  OutDataType=fixdt(1, 16)  OutScaling=2^0  OutDataTypeStr=uint8
  Constant2 : Constant  Value=hex2dec('43')  OutDataTypeMode=uint8  OutDataType=fixdt(1, 16)  OutScaling=2^0  OutDataTypeStr=uint8
  Mux : Mux  Inputs=8
  Out1 : Outport  OutDataType=fixdt(1, 16)  OutScaling=2^0  InitialOutput=[0 0 0 0 0 0 0 0]
  wires:
  Mux/1 -> Out1/1
  Constant1/1 -> Mux/5, Mux/8, Mux/2, Mux/4
  Constant/1 -> Mux/1
  CTR/1 -> Mux/3
  Constant2/1 -> Mux/6, Mux/7

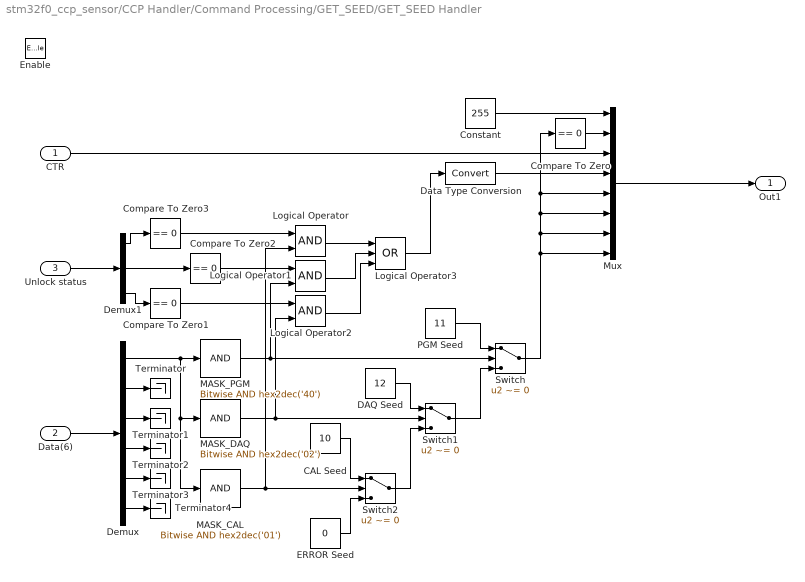
== system stm32f0_ccp_sensor/CCP Handler/Command Processing/GET_SEED/GET_SEED Handler ==
  CTR : Inport  OutDataType=fixdt(1, 16)  OutScaling=2^0
  Data(6) : Inport  Port=2  OutDataType=fixdt(1, 16)  OutScaling=2^0
  Unlock status : Inport  Port=3  OutDataType=fixdt(1, 16)  OutScaling=2^0
  Enable : EnablePort
  CAL Seed : Constant  Value=10  OutDataTypeMode=uint8  OutDataType=fixdt(1, 16)  OutScaling=2^0  OutDataTypeStr=uint8
  Compare To Zero{,1..3} (4 alike) : simulink/Logic and Bit Operations/Compare To Zero  SystemSampleTime=-1  relop===  LogicOutDataTypeMode=uint8  ZeroCross=off
  Constant : Constant  Value=255  OutDataTypeMode=uint8  OutDataType=fixdt(1, 16)  OutScaling=2^0  OutDataTypeStr=uint8
  DAQ Seed : Constant  Value=12  OutDataTypeMode=uint8  OutDataType=fixdt(1, 16)  OutScaling=2^0  OutDataTypeStr=uint8
  Data Type Conversion : DataTypeConversion  OutDataType=fixdt(1, 16)  OutScaling=2^0
  Demux : Demux  Outputs=6
  Demux1 : Demux  Outputs=3
  ERROR Seed : Constant  Value=0  OutDataTypeMode=uint8  OutDataType=fixdt(1, 16)  OutScaling=2^0  OutDataTypeStr=uint8
  Logical Operator : Logic  AllPortsSameDT=off  OutDataTypeMode=boolean  LogicDataType=fixdt(0, 8)  OutDataTypeStr=boolean
  Logical Operator1 : Logic  AllPortsSameDT=off  OutDataTypeMode=boolean  LogicDataType=fixdt(0, 8)  OutDataTypeStr=boolean
  Logical Operator2 : Logic  AllPortsSameDT=off  OutDataTypeMode=boolean  LogicDataType=fixdt(0, 8)  OutDataTypeStr=boolean
  Logical Operator3 : Logic  Operator=OR  Inputs=3  AllPortsSameDT=off  OutDataTypeMode=boolean  LogicDataType=fixdt(0, 8)  OutDataTypeStr=boolean
  MASK_CAL : simulink/Logic and Bit Operations/Bitwise Operator  logicop=AND  UseBitMask=on  BitMask=hex2dec('01')  BitMaskRealWorld=Stored Integer
  MASK_DAQ : simulink/Logic and Bit Operations/Bitwise Operator  logicop=AND  UseBitMask=on  BitMask=hex2dec('02')  BitMaskRealWorld=Stored Integer
  MASK_PGM : simulink/Logic and Bit Operations/Bitwise Operator  logicop=AND  UseBitMask=on  BitMask=hex2dec('40')  BitMaskRealWorld=Stored Integer
  Mux : Mux  Inputs=8
  PGM Seed : Constant  Value=11  OutDataTypeMode=uint8  OutDataType=fixdt(1, 16)  OutScaling=2^0  OutDataTypeStr=uint8
  Switch : Switch  Criteria=u2 ~= 0  OutDataType=fixdt(1, 16)  OutScaling=2^0
  Switch1 : Switch  Criteria=u2 ~= 0  OutDataType=fixdt(1, 16)  OutScaling=2^0
  Switch2 : Switch  Criteria=u2 ~= 0  OutDataType=fixdt(1, 16)  OutScaling=2^0
  Terminator{,1..4} (5 alike) : Terminator
  Out1 : Outport  OutDataType=fixdt(1, 16)  OutScaling=2^0  InitialOutput=[0 0 0 0 0 0 0 0]
  wires:
  CTR/1 -> Mux/3
  Constant/1 -> Mux/1
  Mux/1 -> Out1/1
  Data(6)/1 -> Demux/1
  Demux/1 -> MASK_PGM/1, MASK_DAQ/1, MASK_CAL/1
  MASK_PGM/1 -> Switch/2, Logical Operator1/2
  PGM Seed/1 -> Switch/1
  MASK_DAQ/1 -> Switch1/2, Logical Operator2/2
  DAQ Seed/1 -> Switch1/1
  Switch1/1 -> Switch/3
  MASK_CAL/1 -> Switch2/2, Logical Operator/2
  CAL Seed/1 -> Switch2/1
  Switch2/1 -> Switch1/3
  ERROR Seed/1 -> Switch2/3
  Switch/1 -> Mux/6, Mux/5, Compare To Zero/1, Mux/7, Mux/8
  Demux/2 -> Terminator/1
  Demux/3 -> Terminator1/1
  Demux/4 -> Terminator2/1
  Demux/5 -> Terminator3/1
  Demux/6 -> Terminator4/1
  Compare To Zero/1 -> Mux/2
  Unlock status/1 -> Demux1/1
  Demux1/1 -> Compare To Zero3/1
  Demux1/2 -> Compare To Zero2/1
  Demux1/3 -> Compare To Zero1/1
  Compare To Zero1/1 -> Logical Operator2/1
  Compare To Zero2/1 -> Logical Operator1/1
  Compare To Zero3/1 -> Logical Operator/1
  Logical Operator1/1 -> Logical Operator3/2
  Logical Operator/1 -> Logical Operator3/1
  Logical Operator2/1 -> Logical Operator3/3
  Logical Operator3/1 -> Data Type Conversion/1
  Data Type Conversion/1 -> Mux/4

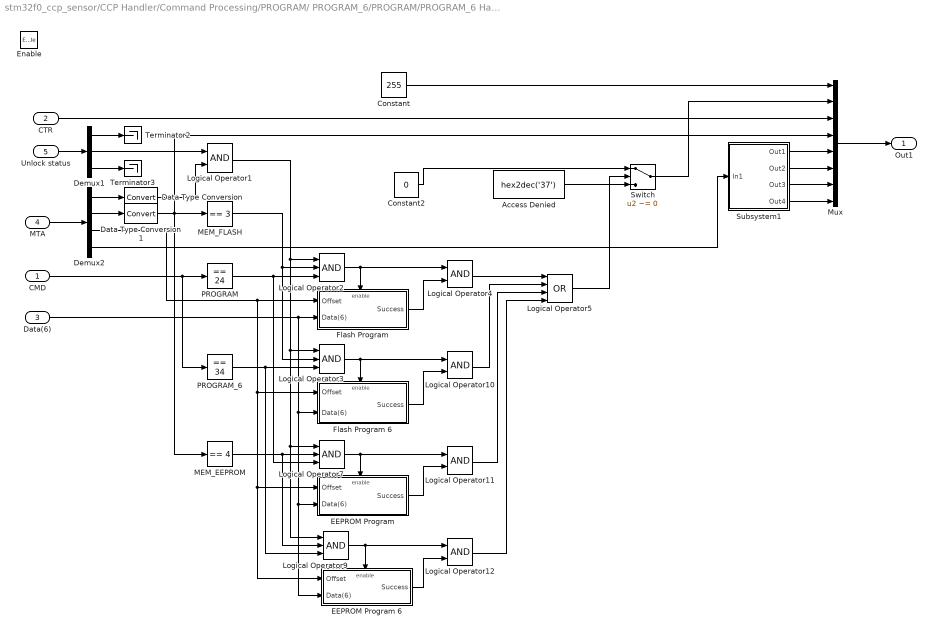
== system stm32f0_ccp_sensor/CCP Handler/Command Processing/PROGRAM/ PROGRAM_6/PROGRAM/PROGRAM_6 Handler ==
  CMD : Inport  OutDataType=fixdt(1, 16)  OutScaling=2^0
  CTR : Inport  Port=2  OutDataType=fixdt(1, 16)  OutScaling=2^0
  Data(6) : Inport  Port=3
  MTA : Inport  Port=4
  Unlock status : Inport  Port=5
  Enable : EnablePort
  Access Denied : Constant  Value=hex2dec('37')  OutDataTypeMode=uint8  OutDataType=fixdt(1, 16)  OutScaling=2^0  OutDataTypeStr=uint8
  Constant : Constant  Value=255  OutDataTypeMode=uint8  OutDataType=fixdt(1, 16)  OutScaling=2^0  OutDataTypeStr=uint8
  Constant2 : Constant  Value=0  OutDataTypeMode=uint8  OutDataType=fixdt(1, 16)  OutScaling=2^0  OutDataTypeStr=uint8
  Data Type Conversion : DataTypeConversion  OutDataType=fixdt(1, 16)  OutScaling=2^0
  Data Type Conversion1 : DataTypeConversion  OutDataType=fixdt(1, 16)  OutScaling=2^0
  Demux1 : Demux  Outputs=3
  Demux2 : Demux
  EEPROM Program : Subsystem
  EEPROM Program 6 : Subsystem
  Flash Program : Subsystem
  Flash Program 6 : Subsystem
  Logical Operator{1,4,10..12} (5 alike) : Logic  AllPortsSameDT=off  OutDataTypeMode=boolean  LogicDataType=fixdt(0, 8)  OutDataTypeStr=boolean
  Logical Operator{2..3,7,9} (4 alike) : Logic  Inputs=3  AllPortsSameDT=off  OutDataTypeMode=boolean  LogicDataType=fixdt(0, 8)  OutDataTypeStr=boolean
  Logical Operator5 : Logic  Operator=OR  Inputs=4  AllPortsSameDT=off  OutDataTypeMode=boolean  LogicDataType=fixdt(0, 8)  OutDataTypeStr=boolean
  MEM_EEPROM : simulink/Logic and Bit Operations/Compare To Constant  SystemSampleTime=-1  relop===  const=4  LogicOutDataTypeMode=uint8  ZeroCross=off
  MEM_FLASH : simulink/Logic and Bit Operations/Compare To Constant  SystemSampleTime=-1  relop===  const=3  LogicOutDataTypeMode=uint8  ZeroCross=off
  Mux : Mux  Inputs=8
  PROGRAM : simulink/Logic and Bit Operations/Compare To Constant  SystemSampleTime=-1  relop===  const=24  LogicOutDataTypeMode=uint8  ZeroCross=off
  PROGRAM_6 : simulink/Logic and Bit Operations/Compare To Constant  SystemSampleTime=-1  relop===  const=34  LogicOutDataTypeMode=uint8  ZeroCross=off
  Subsystem1 : Subsystem
  Switch : Switch  Criteria=u2 ~= 0  OutDataType=fixdt(1, 16)  OutScaling=2^0
  Terminator2 : Terminator
  Terminator3 : Terminator
  Out1 : Outport  OutDataType=fixdt(1, 16)  OutScaling=2^0  InitialOutput=[0 0 0 0 0 0 0 0]
  wires:
  Mux/1 -> Out1/1
  Constant/1 -> Mux/1
  CTR/1 -> Mux/3
  Unlock status/1 -> Demux1/1
  Demux1/1 -> Terminator2/1
  Demux1/3 -> Terminator3/1
  MTA/1 -> Demux2/1
  Switch/1 -> Mux/2
  Subsystem1/1(Out1) -> Mux/5
  Subsystem1/2(Out2) -> Mux/6
  Subsystem1/3(Out3) -> Mux/7
  Subsystem1/4(Out4) -> Mux/8
  Demux2/2 -> Data Type Conversion1/1
  Logical Operator2/1 -> Flash Program/Enable, Logical Operator4/1
  Logical Operator3/1 -> Flash Program 6/Enable, Logical Operator10/1
  Demux2/1 -> Data Type Conversion/1
  Demux1/2 -> Logical Operator1/1
  PROGRAM/1 -> Logical Operator2/3, Logical Operator7/3
  MEM_FLASH/1 -> Logical Operator2/2, Logical Operator3/2
  Logical Operator1/1 -> Logical Operator2/1, Logical Operator3/1, Logical Operator7/1, Logical Operator9/1
  PROGRAM_6/1 -> Logical Operator3/3, Logical Operator9/3
  Logical Operator7/1 -> EEPROM Program/Enable, Logical Operator11/1
  MEM_EEPROM/1 -> Logical Operator7/2, Logical Operator9/2
  Logical Operator9/1 -> EEPROM Program 6/Enable, Logical Operator12/1
  Data(6)/1 -> Flash Program/2(Data(6)), Flash Program 6/2(Data(6)), EEPROM Program/2(Data(6)), EEPROM Program 6/2(Data(6))
  Demux2/3 -> Flash Program/1(Offset), Flash Program 6/1(Offset), EEPROM Program/1(Offset), EEPROM Program 6/1(Offset)
  Demux2/4 -> Subsystem1/1(In1)
  CMD/1 -> PROGRAM/1, PROGRAM_6/1
  Flash Program/1(Success) -> Logical Operator4/2
  Flash Program 6/1(Success) -> Logical Operator10/2
  EEPROM Program/1(Success) -> Logical Operator11/2
  EEPROM Program 6/1(Success) -> Logical Operator12/2
  Logical Operator4/1 -> Logical Operator5/1
  Logical Operator12/1 -> Logical Operator5/4
  Logical Operator11/1 -> Logical Operator5/3
  Logical Operator10/1 -> Logical Operator5/2
  Logical Operator5/1 -> Switch/2
  Access Denied/1 -> Switch/3
  Constant2/1 -> Switch/1
  Data Type Conversion/1 -> Logical Operator1/2
  Data Type Conversion1/1 -> MEM_FLASH/1, MEM_EEPROM/1, Mux/4

== system stm32f0_ccp_sensor/CCP Handler/Command Processing/SET_MTA/SET_MTA Handler ==
  CTR : Inport  OutDataType=fixdt(1, 16)  OutScaling=2^0
  MTA : Inport  Port=2  OutDataType=fixdt(1, 16)  OutScaling=2^0
  Enable : EnablePort
  Constant : Constant  Value=255  OutDataTypeMode=uint8  OutDataType=fixdt(1, 16)  OutScaling=2^0  OutDataTypeStr=uint8
  Constant1 : Constant  Value=0  OutDataTypeMode=uint8  OutDataType=fixdt(1, 16)  OutScaling=2^0  OutDataTypeStr=uint8
  Demux : Demux
  Mux : Mux  Inputs=8
  Out of Range : Constant  Value=hex2dec('32')  OutDataTypeMode=uint8  OutDataType=fixdt(1, 16)  OutScaling=2^0  OutDataTypeStr=uint8
  Switch : Switch  Criteria=u2 ~= 0  OutDataType=fixdt(1, 16)  OutScaling=2^0
  Terminator : Terminator
  Terminator1 : Terminator
  Terminator2 : Terminator
  Out1 : Outport  OutDataType=fixdt(1, 16)  OutScaling=2^0  InitialOutput=[0 0 0 0 0 0 0 0]
  wires:
  Constant1/1 -> Mux/8, Mux/7, Mux/6, Mux/5, Mux/4, Switch/1
  CTR/1 -> Mux/3
  Constant/1 -> Mux/1
  Mux/1 -> Out1/1
  Switch/1 -> Mux/2
  Out of Range/1 -> Switch/3
  MTA/1 -> Demux/1
  Demux/1 -> Switch/2
  Demux/2 -> Terminator/1
  Demux/3 -> Terminator1/1
  Demux/4 -> Terminator2/1

== system stm32f0_ccp_sensor/CCP Handler/Command Processing/SHORT_UP/SHORT_UP Handler ==
  CTR : Inport  OutDataType=fixdt(1, 16)  OutScaling=2^0
  Data(6) : Inport  Port=2  OutDataType=fixdt(1, 16)  OutScaling=2^0
  Enable : EnablePort
  Access Denied : Constant  Value=hex2dec('33')  OutDataTypeMode=uint8  OutDataType=fixdt(1, 16)  OutScaling=2^0  OutDataTypeStr=uint8
  Add : Sum  OutDataType=fixdt(1, 16)  OutScaling=2^-10
  Constant : Constant  Value=255  OutDataTypeMode=uint8  OutDataType=fixdt(1, 16)  OutScaling=2^0  OutDataTypeStr=uint8
  Constant1 : Constant  Value=0  OutDataTypeMode=uint8  OutDataType=fixdt(1, 16)  OutScaling=2^0  OutDataTypeStr=uint8
  Data Type Conversion : DataTypeConversion  OutDataType=fixdt(1, 16)  OutScaling=2^0
  Demux : Demux  Outputs=6
  Demux2 : Demux  Outputs=5
  Interval Test1 : simulink/Logic and Bit Operations/Interval Test  SystemSampleTime=-1  IntervalClosedRight=on  uplimit=5  IntervalClosedLeft=on  lowlimit=1  LogicOutDataTypeMode=boolean
  Logical Operator1 : Logic  AllPortsSameDT=off  OutDataTypeMode=boolean  LogicDataType=fixdt(0, 8)  OutDataTypeStr=boolean
  Mux : Mux  Inputs=8
  Out of Range : Constant  Value=hex2dec('33')  OutDataTypeMode=uint8  OutDataType=fixdt(1, 16)  OutScaling=2^0  OutDataTypeStr=uint8
  Subsystem : Subsystem
  Switch1 : Switch  Criteria=u2 ~= 0  OutDataType=fixdt(1, 16)  OutScaling=2^0
  Switch2 : Switch  Criteria=u2 ~= 0  OutDataType=fixdt(1, 16)  OutScaling=2^0
  UPLOAD : Subsystem
  Validate Base Address : Subsystem
  Out1 : Outport  OutDataType=fixdt(1, 16)  OutScaling=2^0  InitialOutput=[0 0 0 0 0 0 0 0]
  wires:
  Demux/1 -> Data Type Conversion/1, Interval Test1/1, Add/1
  Data(6)/1 -> Demux/1
  CTR/1 -> Mux/3
  Constant/1 -> Mux/1
  Mux/1 -> Out1/1
  Out of Range/1 -> Switch1/3
  Switch2/1 -> Switch1/1
  Access Denied/1 -> Switch2/3
  Constant1/1 -> Switch2/1
  Demux2/1 -> Mux/4
  Demux2/2 -> Mux/5
  Demux2/3 -> Mux/6
  Demux2/4 -> Mux/7
  Demux2/5 -> Mux/8
  Data Type Conversion/1 -> UPLOAD/3(Size)
  Switch1/1 -> Mux/2
  Interval Test1/1 -> Logical Operator1/2
  Logical Operator1/1 -> Switch1/2, UPLOAD/Enable
  UPLOAD/2(Out1) -> Demux2/1
  UPLOAD/1(Valid) -> Switch2/2
  Demux/2 -> Validate Base Address/1(ExtAddr), UPLOAD/1(Mem Sector)
  Validate Base Address/1(ValidAddr) -> Logical Operator1/1
  Demux/3 -> Subsystem/1(In1)
  Demux/4 -> Subsystem/2(In2)
  Demux/5 -> Subsystem/3(In3)
  Demux/6 -> Subsystem/4(In4)
  Subsystem/1(Out1) -> Add/2, UPLOAD/2(Offset)
  Add/1 -> Validate Base Address/2(PostIncAddr)

== system stm32f0_ccp_sensor/CCP Handler/Command Processing/UNLOCK/UNLOCK Handler ==
  CTR : Inport  OutDataType=fixdt(1, 16)  OutScaling=2^0
  Unlock status : Inport  Port=2  OutDataType=fixdt(1, 16)  OutScaling=2^0
  Enable : EnablePort
  Bitwise Operator : simulink/Logic and Bit Operations/Bitwise Operator  logicop=OR  UseBitMask=off  NumInputPorts=3  BitMask=bin2dec('11011001')  BitMaskRealWorld=Stored Integer
  Constant : Constant  Value=255  OutDataTypeMode=uint8  OutDataType=fixdt(1, 16)  OutScaling=2^0  OutDataTypeStr=uint8
  Constant1 : Constant  Value=0  OutDataTypeMode=uint8  OutDataType=fixdt(1, 16)  OutScaling=2^0  OutDataTypeStr=uint8
  Constant2 : Constant  Value=0  OutDataTypeMode=uint8  OutDataType=fixdt(1, 16)  OutScaling=2^0  OutDataTypeStr=uint8
  Data Type Conversion : DataTypeConversion  OutDataType=fixdt(1, 16)  OutScaling=2^0
  Demux : Demux  Outputs=3
  Mask CAL : Constant  Value=hex2dec('01')  OutDataTypeMode=uint8  OutDataType=fixdt(1, 16)  OutScaling=2^0  OutDataTypeStr=uint8
  Mask DAQ : Constant  Value=hex2dec('02')  OutDataTypeMode=uint8  OutDataType=fixdt(1, 16)  OutScaling=2^0  OutDataTypeStr=uint8
  Mask PGM : Constant  Value=hex2dec('40')  OutDataTypeMode=uint8  OutDataType=fixdt(1, 16)  OutScaling=2^0  OutDataTypeStr=uint8
  Mux : Mux  Inputs=8
  Switch1 : Switch  Criteria=u2 ~= 0  OutDataType=fixdt(1, 16)  OutScaling=2^0
  Switch2 : Switch  Criteria=u2 ~= 0  OutDataType=fixdt(1, 16)  OutScaling=2^0
  Switch3 : Switch  Criteria=u2 ~= 0  OutDataType=fixdt(1, 16)  OutScaling=2^0
  Out1 : Outport  OutDataType=fixdt(1, 16)  OutScaling=2^0  InitialOutput=[0 0 0 0 0 0 0 0]
  wires:
  Mux/1 -> Out1/1
  Constant/1 -> Mux/1
  CTR/1 -> Mux/3
  Unlock status/1 -> Demux/1
  Constant1/1 -> Mux/2, Mux/5, Mux/6, Mux/7, Mux/8
  Demux/1 -> Switch1/2
  Demux/2 -> Switch2/2
  Demux/3 -> Switch3/2
  Mask CAL/1 -> Switch1/1
  Mask PGM/1 -> Switch2/1
  Mask DAQ/1 -> Switch3/1
  Constant2/1 -> Switch3/3, Switch2/3, Switch1/3
  Switch1/1 -> Bitwise Operator/1
  Switch2/1 -> Bitwise Operator/2
  Switch3/1 -> Bitwise Operator/3
  Data Type Conversion/1 -> Mux/4
  Bitwise Operator/1 -> Data Type Conversion/1
